simulink model "uloha3"  (Simulink 7.5)
settings: Solver=ode45  StartTime=0.0  StopTime=10.0  RelTol=1e-3
settings Model: Creator=michal  LastModifiedBy=michal

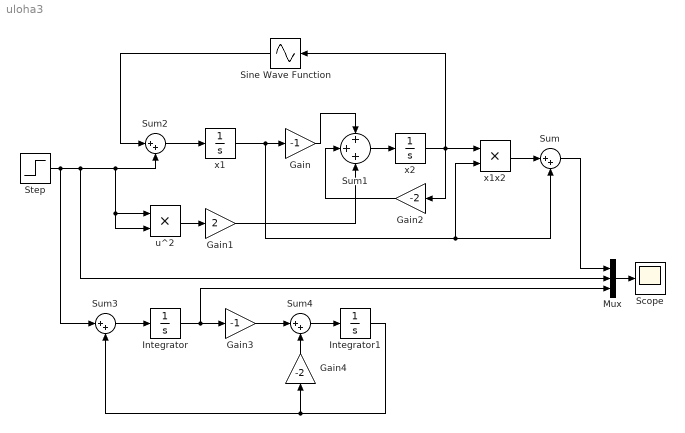
== system uloha3 ==
  Gain : Gain  Gain=-1  ParameterDataType=fixdt(1, 16)  ParameterScaling=2^0  OutDataType=fixdt(1, 16)  OutScaling=2^0
  Gain1 : Gain  Gain=2  ParameterDataType=fixdt(1, 16)  ParameterScaling=2^0  OutDataType=fixdt(1, 16)  OutScaling=2^0
  Gain2 : Gain  Gain=-2  ParameterDataType=fixdt(1, 16)  ParameterScaling=2^0  OutDataType=fixdt(1, 16)  OutScaling=2^0
  Gain3 : Gain  Gain=-1  ParameterDataType=fixdt(1, 16)  ParameterScaling=2^0  OutDataType=fixdt(1, 16)  OutScaling=2^0
  Gain4 : Gain  Gain=-2  ParameterDataType=fixdt(1, 16)  ParameterScaling=2^0  OutDataType=fixdt(1, 16)  OutScaling=2^0
  Integrator : Integrator
  Integrator1 : Integrator
  Mux : Mux  Inputs=3
  Scope : Scope
      settings: AttributesFormatString=%<AxesTitles>  SaveName=nestab  DataFormat=Array
  Sine Wave Function : Sin  TimeSource=Use external signal  Amplitude=1  Bias=0  Frequency=1  Phase=0  Samples=10  SampleTime=0  Offset=0
  Step : Step  After=0.5  SampleTime=0
  Sum{,2..4} (4 alike) : Sum  Inputs=|++  OutDataType=fixdt(1, 16)  OutScaling=2^0
  Sum1 : Sum  Inputs=+++  OutDataType=fixdt(1, 16)  OutScaling=2^0
  u^2 : Product  OutDataType=fixdt(1, 16)  OutScaling=2^0  RndMeth=Zero
  x1 : Integrator
  x1x2 : Product  OutDataType=fixdt(1, 16)  OutScaling=2^0  RndMeth=Zero
  x2 : Integrator
  wires:
  x1x2/1 -> Sum/1
  x2/1 -> x1x2/1, Gain2/1, Sine Wave Function/1
  x1/1 -> Gain/1, x1x2/2, Sum/2
  Sum1/1 -> x2/1
  Sum2/1 -> x1/1
  Sine Wave Function/1 -> Sum2/1
  Step/1 -> Sum3/1, Sum2/2, u^2/1, u^2/2, Mux/2
  Gain/1 -> Sum1/1
  u^2/1 -> Gain1/1
  Gain1/1 -> Sum1/3
  Gain2/1 -> Sum1/2
  Sum3/1 -> Integrator/1
  Integrator1/1 -> Sum3/2, Gain4/1
  Gain3/1 -> Sum4/1
  Integrator/1 -> Gain3/1, Mux/3
  Gain4/1 -> Sum4/2
  Sum4/1 -> Integrator1/1
  Mux/1 -> Scope/1
  Sum/1 -> Mux/1
